simulink model "gpt_rdf4_angle"  (R2013b)
settings: Solver=FixedStepDiscrete  StartTime=0.0  StopTime=4  FixedStep=1/800  RelTol=1e-3
libraries: commanapbnd3 x5
settings Model: Creator=rmg37  LastModifiedBy=rmg37
settings DataIOCC: SaveOutput=off  SaveTime=off
settings OptimizationCC: LocalBlockOutputs=off
settings DebuggingCC: AlgebraicLoopMsg=error  SingleTaskRateTransMsg=error

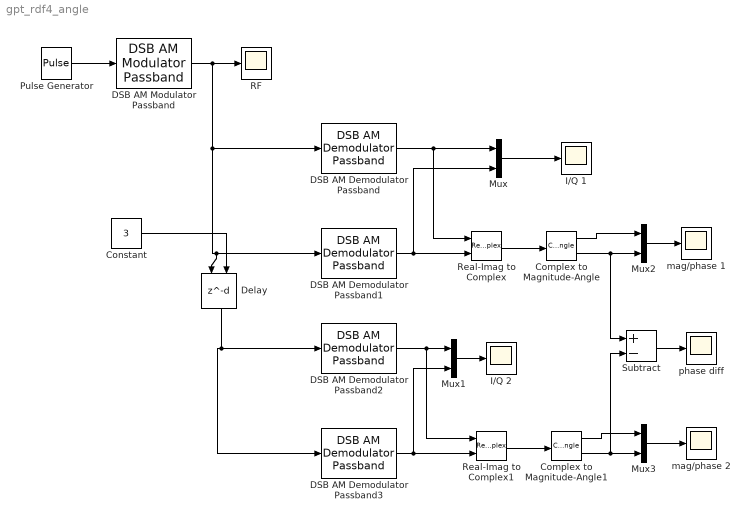
== system gpt_rdf4_angle ==
  Complex to Magnitude-Angle : ComplexToMagnitudeAngle
  Complex to Magnitude-Angle1 : ComplexToMagnitudeAngle
  Constant : Constant  Value=3
  DSB AM Demodulator Passband : commanapbnd3/DSB AM Demodulator Passband  Fc=100  Ph=0  method=Butterworth  n=4  cf=4  Rp=0.1  Rs=50  Offset=0
  DSB AM Demodulator Passband1 : commanapbnd3/DSB AM Demodulator Passband  Fc=100  Ph=pi/2  method=Butterworth  n=4  cf=4  Rp=0.1  Rs=50  Offset=0
  DSB AM Demodulator Passband2 : commanapbnd3/DSB AM Demodulator Passband  Fc=100  Ph=0  method=Butterworth  n=4  cf=4  Rp=0.1  Rs=50  Offset=0
  DSB AM Demodulator Passband3 : commanapbnd3/DSB AM Demodulator Passband  Fc=100  Ph=pi/2  method=Butterworth  n=4  cf=4  Rp=0.1  Rs=50  Offset=0
  DSB AM Modulator Passband : commanapbnd3/DSB AM Modulator Passband  Fc=99.9  Ph=0  Offset=0
  Delay : Delay  DelayLengthSource=Input port
      settings: InputPortMap=u0,p1
  I/Q 1 : Scope
  I/Q 2 : Scope
      settings: SaveName=ScopeData2
  Mux{,1..3} (4 alike) : Mux  Inputs=2
  Pulse Generator : DiscretePulseGenerator  PulseType=Time based  PulseWidth=50
  RF : Scope
      settings: Tag=RF waveform
  Real-Imag to Complex : RealImagToComplex
  Real-Imag to Complex1 : RealImagToComplex
  Subtract : Sum  Inputs=+-
  mag/phase 1 : Scope
      settings: SaveName=ScopeData3
  mag/phase 2 : Scope
      settings: SaveName=ScopeData4
  phase diff : Scope
      settings: SaveName=ScopeData5
  wires:
  Pulse Generator/1 -> DSB AM Modulator Passband/1
  DSB AM Demodulator Passband/1 -> Real-Imag to Complex/1, Mux/1
  Mux/1 -> I/Q 1/1
  DSB AM Demodulator Passband1/1 -> Mux/2, Real-Imag to Complex/2
  DSB AM Modulator Passband/1 -> Delay/1, DSB AM Demodulator Passband1/1, DSB AM Demodulator Passband/1, RF/1
  DSB AM Demodulator Passband2/1 -> Real-Imag to Complex1/1, Mux1/1
  Mux1/1 -> I/Q 2/1
  DSB AM Demodulator Passband3/1 -> Mux1/2, Real-Imag to Complex1/2
  Real-Imag to Complex/1 -> Complex to Magnitude-Angle/1
  Mux2/1 -> mag/phase 1/1
  Complex to Magnitude-Angle/2 -> Subtract/1, Mux2/2
  Complex to Magnitude-Angle/1 -> Mux2/1
  Real-Imag to Complex1/1 -> Complex to Magnitude-Angle1/1
  Mux3/1 -> mag/phase 2/1
  Complex to Magnitude-Angle1/2 -> Subtract/2, Mux3/2
  Complex to Magnitude-Angle1/1 -> Mux3/1
  Subtract/1 -> phase diff/1
  Delay/1 -> DSB AM Demodulator Passband3/1, DSB AM Demodulator Passband2/1
  Constant/1 -> Delay/2
